simulink model "tqdtqr_rebuild_V3"  (R2021b)
settings: Solver=VariableStepAuto  StartTime=0.0  StopTime=10.0  RelTol=1e-3
undefined symbols (not defined in the file): ATQD_AfterTqMinGain_X_Deg, ATQD_APSCreepBaseTqD_X_kph, ATQD_APSCreepBaseTqD_Y_Deg, ATQD_APSCreepBaseTqR_X_kph, ATQD_APSCreepBaseTqR_Y_Deg, ATQD_APSCreepIterm_X_kph, ATQD_APSCreepIterm_Y_kph, ATQD_APSCreepPterm_X_kph, ATQD_APSCreepPterm_Y_kph, ATQD_APSDecReq_X_kph, ATQD_APSDecReq_Y_mps2, ATQD_APSDecReqCMD_X_kph, ATQD_APSDecReqTs_X_pct, ATQD_APSDecTimeGain_X_Deg, ATQD_APSDecTimeGain_Y_s, ATQD_APSReqLowSpd_X_Deg, ATQD_AutoHoldReleaseBPS_X_Deg, ATQD_AWDLoadTrqnsGain_X_kg, ATQD_AWDLoadTrqnsGain_Y_pct, ATQD_BOSEnBPSPosn_X_kph, ATQD_BOSMap_X_rpm, ATQD_BOSMap_Y_pct, ATQD_CreepBaseTqD_X_kph, ATQD_CreepBaseTqD_Y_Deg, ATQD_CreepBaseTqR_X_kph, ATQD_CreepBaseTqR_Y_Deg, ATQD_CreepBPSDisPosn_X_Deg, ATQD_CreepBPSDisPosnR_X_Deg, ATQD_CreepBPSEnPosn_X_Deg, ATQD_CreepBPSEnPosnR_X_Deg, ATQD_CreepDeltaTq_X_kph, ATQD_CreepIterm_X_kph, ATQD_CreepIterm_Y_kph, ATQD_CreepItermMaxLimit_X_pct, ATQD_CreepPreloadTime_X_kph, ATQD_CreepPreloadTq_X_kph, ATQD_CreepPreloadTq_Y_s, ATQD_CreepProtTq_X_Deg, ATQD_CreepPterm_X_kph, ATQD_CreepPterm_Y_kph, ATQD_CreepRrTqSpRat_X_rpm, ATQD_CreepRrTqSpRat_Y_Nm, ATQD_CreepTargetSpdD_X_pct, ATQD_CreepTargetSpdR_X_pct, ATQD_CreepUpLimitTq_X_rpm, ATQD_DecIneOPDHoldEnDelay_X_Deg, ATQD_DecIneOPDHoldEnDelay_Y_bar, ATQD_ECOTqMapD_X_rpm, ATQD_ECOTqMapD_Y_pct, ATQD_EMTqMapD_X_rpm, ATQD_EMTqMapD_Y_pct, ATQD_EOPDTqMapDCon_X_rpm, ATQD_EOPDTqMapDCon_Y_Deg, ATQD_EstInitVehWeight_X_c, ATQD_FAfterTqCMDGain_X_rpm, ATQD_FAfterTqCMDGain_Y_pct, ATQD_ForceLowSpd_X_Deg, ATQD_ForcePLimitSpd_X_Deg, ATQD_FrLossMAPLowV_X_rpm, ATQD_FrLossMAPLowV_Y_Nm ... (+949)
libraries: simulink x235, hcu_lib x208, tqr x63, tqd x6
(part 9 of 37)

== system tqdtqr_rebuild_V3/Input_Convert/Main function/Add B regen to ramp enable judge ==
  note: Rear B regen
  note: Front B regen
  BSCPIn_outputs : Inport
  BSignalConvert_outputs : Inport  Port=2
  BFunction_outputs : Inport  Port=3
  AND{6..7,10,12} (4 alike) : Logic  AllPortsSameDT=off  OutDataTypeStr=boolean
  AND{8..9,11,13} (4 alike) : Logic  Operator=OR  AllPortsSameDT=off  OutDataTypeStr=boolean
  AND{3,5,14,16} (4 alike) : Logic  Inputs=3  AllPortsSameDT=off  OutDataTypeStr=boolean
  AND15 : Logic  Operator=OR  Inputs=3  AllPortsSameDT=off  OutDataTypeStr=boolean
  AND17 : Logic  Operator=OR  Inputs=3  AllPortsSameDT=off  OutDataTypeStr=boolean
  Add2 : Sum
  Add3 : Sum
  Bus Selector : BusSelector  OutputSignals=task_time_s,VVMC_ADASActive_flg,VINP_FrntAxlTrqReqBrk_Nm,VINP_FrRBCActive_flg,VINP_RearAxlTrqReqBrk_Nm,VINP_RrRBCActive_flg
  Bus Selector1 : BusSelector  OutputSignals=VTQD_BrkSwSta_flg,VTQR_RampTqCMDGain_c
  Bus Selector2 : BusSelector  OutputSignals=VTQD_GearActualPosn_enum
  Constant14 : Constant  Value=ONE_INT
  Constant15 : Constant  Value=KTQR_NewRampArchSW_flg
  Constant22 : Constant  Value=ONE_INT
  Constant23 : Constant  Value=ENUM_GEARACTUALPOSN_R
  Constant30 : Constant  Value=KTQR_NewRampArchSW_flg
  Constant31 : Constant  Value=ENUM_GEARACTUALPOSN_R
  Constant32 : Constant  Value=KTQR_ACCCancelNoRBC_flg
  Constant33 : Constant  Value=KTQR_ACCCancelNoRBC_flg
  Constant{4..5,34,39} (4 alike) : Constant  Value=ZERO_FLOAT
  Constant35 : Constant  Value=KTQR_ADASCancelBRgnSlopeF_Nmps
  Constant{36..38,41} (4 alike) : Constant  Value=KTQR_ADASCancelBRgnSlopeSW_flg
  Constant40 : Constant  Value=KTQR_ADASCancelBRgnSlopeR_Nmps
  Detect Decrease{,1..3} (4 alike) : simulink/Logic and Bit Operations/Detect Decrease  vinit=0.0  OutDataTypeStr=boolean
  Divide : Product  Inputs=**
  Divide1 : Product  Inputs=**
  Equal8 : RelationalOperator  Operator===  OutDataTypeStr=boolean  RndMeth=Simplest
  Equal9 : RelationalOperator  Operator===  OutDataTypeStr=boolean  RndMeth=Simplest
  NOT{,1..11} (12 alike) : Logic  Operator=NOT  AllPortsSameDT=off  OutDataTypeStr=boolean
  Product2 : Product
  Product5 : Product
  Relational Operator : RelationalOperator  Operator=<=  OutDataTypeStr=boolean  RndMeth=Simplest
  Relational Operator1 : RelationalOperator  Operator=<=  OutDataTypeStr=boolean  RndMeth=Simplest
  SR_Latch{1..4} (4 alike) : hcu_lib/Basic_Blocks/SR_Latch
  Switch{4..5,12,17,22..27} (10 alike) : Switch  Criteria=u2 ~= 0
      settings: AttributesFormatString=%<Criteria>
  Unit Delay{,1..3} (4 alike) : UnitDelay  InitialCondition=single(0)  SampleTime=-1  HasFrameUpgradeWarning=on
      settings: AttributesFormatString=%<InitialCondition>
  VTQD_FEDUWhlTqBRegen_Nm : Outport
  VTQD_REDUWhlTqBRegen_Nm : Outport  Port=2
  wires:
  [VTQD_BrkSwSta_flg] -> AND14/2
  [task_time_s] -> Divide/2
  [VVMC_ADASActive_flg] -> Detect Decrease2/1
  Constant36/1 -> AND14/3
  Divide/1 -> Add2/2
  [VINP_FrRBCActive_flg] -> NOT9/1
  SR_Latch3/1 -> [VTQR_ADASCancelBRgnRampF_flg]  "VTQR_ADASCancelBRgnRampF_flg"
  [VTQD_BrkSwSta_flg] -> NOT8/1
  [VTQR_FrntAxlTrqReqBrkRamp_Nm] -> Unit Delay2/1
  [VINP_FrntAxlTrqReqBrk_Nm] -> Relational Operator/2
  Unit Delay2/1 -> Relational Operator/1
  NOT8/1 -> AND15/2
  [VTQR_ADASCancelBRgnRampF_flg] -> Switch22/2
  Detect Decrease2/1 -> AND14/1
  Unit Delay/1 -> Add2/1
  AND14/1 -> SR_Latch3/1
  AND15/1 -> SR_Latch3/2
  Relational Operator/1 -> AND15/1
  Switch22/1 -> Unit Delay/1, [VTQR_FrntAxlTrqReqBrkRamp_Nm]  "VTQR_FrntAxlTrqReqBrkRamp_Nm"
  Constant35/1 -> Divide/1
  Constant34/1 -> Switch22/3
  Add2/1 -> Switch22/1
  NOT9/1 -> AND15/3
  [VINP_FrRBCActive_flg] -> AND3/3
  [VVMC_ADASActive_flg] -> NOT1/1
  [VINP_FrntAxlTrqReqBrk_Nm] -> Switch26/3
  [VTQR_RampTqCMDGain_c] -> Switch12/1
  NOT1/1 -> AND3/1
  Switch26/1 -> Switch23/1
  AND13/1 -> SR_Latch2/2
  NOT3/1 -> AND8/2
  Constant30/1 -> AND7/2
  AND12/1 -> SR_Latch2/1
  [VVMC_ADASActive_flg] -> Detect Decrease1/1
  [VTQD_BrkSwSta_flg] -> NOT5/1
  AND3/1 -> Switch4/2
  AND7/1 -> Switch12/2
  AND8/1 -> AND3/2
  Equal9/1 -> AND7/1
  Constant31/1 -> Equal9/2
  Constant4/1 -> Switch4/3
  Constant32/1 -> NOT3/1
  [VTQD_GearActualPosn_enum] -> Equal9/1
  [VTQR_FrntAxlTrqReqBrkRamp_Nm] -> Switch26/1
  SR_Latch2/1 -> NOT7/1
  [VTQR_ADASCancelBRgnRampF_flg] -> Switch26/2
  [VINP_FrntAxlTrqReqBrk_Nm] -> Switch23/3
  Switch23/1 -> Switch4/1
  [VVMC_ADASActive_flg] -> AND13/1
  [VTQD_BrkSwSta_flg] -> AND13/2
  Detect Decrease1/1 -> AND12/1
  Switch12/1 -> Product2/2
  NOT5/1 -> AND12/2
  Switch4/1 -> Product2/1
  Constant37/1 -> Switch23/2
  NOT7/1 -> AND8/1
  Constant14/1 -> Switch12/3
  BSCPIn_outputs/1 -> Bus Selector/1
  Bus Selector/2 -> [VVMC_ADASActive_flg]  "<VVMC_ADASActive_flg>"
  Bus Selector/3 -> [VINP_FrntAxlTrqReqBrk_Nm]  "<VINP_FrntAxlTrqReqBrk_Nm>"
  Bus Selector/4 -> [VINP_FrRBCActive_flg]  "<VINP_FrRBCActive_flg>"
  Bus Selector/1 -> [task_time_s]  "<task_time_s>"
  BSignalConvert_outputs/1 -> Bus Selector1/1
  BFunction_outputs/1 -> Bus Selector2/1
  Bus Selector1/1 -> [VTQD_BrkSwSta_flg]  "<VTQD_BrkSwSta_flg>"
  Bus Selector2/1 -> [VTQD_GearActualPosn_enum]  "<VTQD_GearActualPosn_enum>"
  Bus Selector1/2 -> [VTQR_RampTqCMDGain_c]  "<VTQR_RampTqCMDGain_c>"
  Product2/1 -> [VTQD_FEDUWhlTqBRegen_Nm]  "VTQD_FEDUWhlTqBRegen_Nm"
  [VTQD_FEDUWhlTqBRegen_Nm] -> VTQD_FEDUWhlTqBRegen_Nm/1
  Relational Operator1/1 -> AND17/1
  [VINP_RrRBCActive_flg] -> NOT11/1
  [VINP_RearAxlTrqReqBrk_Nm] -> Relational Operator1/2
  Detect Decrease3/1 -> AND16/1
  [VTQD_BrkSwSta_flg] -> NOT10/1
  Divide1/1 -> Add3/2
  [VVMC_ADASActive_flg] -> Detect Decrease3/1
  [VTQR_ADASCancelBRgnRampR_flg] -> Switch25/2
  Switch25/1 -> Unit Delay1/1, [VTQR_RearAxlTrqReqBrkRamp_Nm]  "VTQR_RearAxlTrqReqBrkRamp_Nm"
  Unit Delay3/1 -> Relational Operator1/1
  AND17/1 -> SR_Latch4/2
  [VTQR_RearAxlTrqReqBrkRamp_Nm] -> Unit Delay3/1
  NOT11/1 -> AND17/3
  NOT10/1 -> AND17/2
  Add3/1 -> Switch25/1
  SR_Latch4/1 -> [VTQR_ADASCancelBRgnRampR_flg]  "VTQR_ADASCancelBRgnRampR_flg"
  Unit Delay1/1 -> Add3/1
  Constant39/1 -> Switch25/3
  Constant41/1 -> AND16/3
  Constant40/1 -> Divide1/1
  [VTQD_BrkSwSta_flg] -> AND16/2
  AND16/1 -> SR_Latch4/1
  [task_time_s] -> Divide1/2
  Constant22/1 -> Switch17/3
  [VTQR_RampTqCMDGain_c] -> Switch17/1
  [VVMC_ADASActive_flg] -> NOT2/1
  AND5/1 -> Switch5/2
  NOT2/1 -> AND5/1
  Constant5/1 -> Switch5/3
  [VVMC_ADASActive_flg] -> Detect Decrease/1
  Switch5/1 -> Product5/1
  [VINP_RearAxlTrqReqBrk_Nm] -> Switch24/3
  [VINP_RrRBCActive_flg] -> AND5/3
  [VTQR_RearAxlTrqReqBrkRamp_Nm] -> Switch27/1
  [VTQD_BrkSwSta_flg] -> NOT/1
  [VTQD_BrkSwSta_flg] -> AND11/2
  Detect Decrease/1 -> AND10/1
  [VTQD_GearActualPosn_enum] -> Equal8/1
  AND10/1 -> SR_Latch1/1
  Constant15/1 -> AND6/2
  Equal8/1 -> AND6/1
  Switch17/1 -> Product5/2
  AND11/1 -> SR_Latch1/2
  [VTQR_ADASCancelBRgnRampR_flg] -> Switch27/2
  Switch27/1 -> Switch24/1
  Constant23/1 -> Equal8/2
  [VINP_RearAxlTrqReqBrk_Nm] -> Switch27/3
  Constant38/1 -> Switch24/2
  NOT4/1 -> AND9/2
  AND6/1 -> Switch17/2
  NOT6/1 -> AND9/1
  Constant33/1 -> NOT4/1
  [VVMC_ADASActive_flg] -> AND11/1
  NOT/1 -> AND10/2
  SR_Latch1/1 -> NOT6/1
  AND9/1 -> AND5/2
  Switch24/1 -> Switch5/1
  Product5/1 -> [VTQD_REDUWhlTqBRegen_Nm]  "VTQD_REDUWhlTqBRegen_Nm"
  [VTQD_REDUWhlTqBRegen_Nm] -> VTQD_REDUWhlTqBRegen_Nm/1
  Bus Selector/5 -> [VINP_RearAxlTrqReqBrk_Nm]  "<VINP_RearAxlTrqReqBrk_Nm>"
  Bus Selector/6 -> [VINP_RrRBCActive_flg]  "<VINP_RrRBCActive_flg>"

== system tqdtqr_rebuild_V3/Input_Convert/Main function/AvaliableTqLimit function ==
  BSCPIn_outputs : Inport
  BSignalConvert_outputs : Inport  Port=2
  BFunction_outputs : Inport  Port=3
  BMain_outputs : Inport  Port=4
  VTQD_IVIRockModeEn_flg : Inport  Port=5
  VTQD_FrEDUSpRat_rat : Inport  Port=6
  VTQD_RrEDUSpRat_rat : Inport  Port=7
  Bus Selector : BusSelector  OutputSignals=task_time_s,VINP_HVBPwrAvailDchrg_kW,VINP_HVBPwrAvailChrg_kW,VINP_FrMotorAvailTq_Nm,VINP_RrMotorAvailTq_Nm,VINP_FrRegenAvailTq_Nm,VINP_RrRegenAvailTq_Nm,VINP_VehicleType_enum,VINP_FrMCUDCBusVolt_V,VINP_RrMCUDCBusVolt_V,VPMM_DrivetrainSelect_enum,VINP_FrMCUTemp_C,VINP_FrTMTemp_C,VINP_RrMCUTemp_C,VINP_RrTMTemp_C,VVMC_EstSlope_Deg,VINP_FrPTCSActive_flg,VINP_RrPTCSActive_flg,VTQD_ActAPSPosn_pct
  Bus Selector1 : BusSelector  OutputSignals=VTQD_FrShaftSpd_rpm,VTQD_RrShaftSpd_rpm
  Bus Selector2 : BusSelector  OutputSignals=VTQD_GearActualPosn_enum,VTQD_FrontSlideRate_pct,VTQD_RearSlideRate_pct
  Bus Selector4 : BusSelector  OutputSignals=VTQD_CoordWhlTqDemFr_Nm,VTQD_CoordWhlTqDemRr_Nm
  Constant2 : Constant  Value=KTQD_FrBatapCont_factor
  Constant{27,30,51..52} (4 alike) : Constant  Value=ONE_FLOAT
  Constant28 : Constant  Value=KTQD_FAfterTqCMDGainInc_c
  Constant29 : Constant  Value=KTQD_FAfterTqCMDGainDec_c
  Constant31 : Constant  Value=KTQD_RAfterTqCMDGainInc_c
  Constant32 : Constant  Value=KTQD_RAfterTqCMDGainDec_c
  Constant5 : Constant  Value=KTQD_RrBatapCont_factor
  MTQD_AfterTqMinGain_Y_c : Lookup_n-D  NumberOfTableDimensions=1  BreakpointsForDimension1=ATQD_AfterTqMinGain_X_Deg  Table=MTQD_AfterTqMinGain_Y_c  InternalRulePriority=Speed  RndMeth=Simplest  InputSameDT=on
  MTQD_FAfterTqCMDGain_Z_c : Lookup_n-D  BreakpointsForDimension1=ATQD_FAfterTqCMDGain_Y_pct  BreakpointsForDimension2=ATQD_FAfterTqCMDGain_X_rpm  Table=MTQD_FAfterTqCMDGain_Z_c  InternalRulePriority=Speed  RndMeth=Simplest  InputSameDT=on
      settings: InputPortMap=u0,u1
  MTQD_RAfterTqCMDGain_Z_c : Lookup_n-D  BreakpointsForDimension1=ATQD_FAfterTqCMDGain_Y_pct  BreakpointsForDimension2=ATQD_FAfterTqCMDGain_X_rpm  Table=MTQD_RAfterTqCMDGain_Z_c  InternalRulePriority=Speed  RndMeth=Simplest  InputSameDT=on
      settings: InputPortMap=u0,u1
  Max2 : MinMax  Function=max  Inputs=2
  Max3 : MinMax  Function=max  Inputs=2
  RateLimit : hcu_lib/Basic_Blocks/RateLimit
  RateLimit1 : hcu_lib/Basic_Blocks/RateLimit
  Switch13 : Switch  Criteria=u2 > Threshold
  Switch14 : Switch  Criteria=u2 > Threshold
  TorqueCapacityCalcalation : Subsystem
  VTQD_WhlTqCapMotFr_Nm : Outport
  VTQD_WhlTqCapMotRr_Nm : Outport  Port=2
  VTQD_WhlTqCapGenFr_Nm : Outport  Port=3
  VTQD_WhlTqCapGenRr_Nm : Outport  Port=4
  VTQD_MotorLossTotal_kw : Outport  Port=5
  VTQD_FAfterTqCMDGain_c : Outport  Port=6
  VTQD_RAfterTqCMDGain_c : Outport  Port=7
  wires:
  TorqueCapacityCalcalation/5(VTQD_MotorLossTotal_kw) -> [VTQD_MotorLossTotal_kw]
  [VINP_RrMCUTemp_C] -> TorqueCapacityCalcalation/22(VINP_RrMCUTemp_C)
  TorqueCapacityCalcalation/3(VTQD_WhlTqCapGenFr_Nm) -> [VTQD_WhlTqCapGenFr_Nm]
  [VINP_FrTMTemp_C] -> TorqueCapacityCalcalation/21(VINP_FrTMTemp_C)
  [VINP_FrMCUTemp_C] -> TorqueCapacityCalcalation/20(VINP_FrMCUTemp_C)
  [VPMM_DrivetrainSelect_enum] -> TorqueCapacityCalcalation/19(VPMM_DrivetrainSelect_enum)
  [VTQD_CoordWhlTqDemFr_Nm] -> TorqueCapacityCalcalation/15(VTQD_CoordWhlTqDemFr_Nm)
  [VTQD_RrEDUSpRat_rat] -> TorqueCapacityCalcalation/8(VTQD_RrEDUSpRat_rat)
  [VINP_FrRegenAvailTq_Nm] -> TorqueCapacityCalcalation/11(VINP_FrRegenAvailTq_Nm)
  Constant5/1 -> TorqueCapacityCalcalation/6(KTQD_RrBatapCont_factor)
  Constant2/1 -> TorqueCapacityCalcalation/5(KTQD_FrBatapCont_factor)
  [VINP_RrTMTemp_C] -> TorqueCapacityCalcalation/23(VINP_RrTMTemp_C)
  TorqueCapacityCalcalation/1(VTQD_WhlTqCapMotFr_Nm) -> [VTQD_WhlTqCapMotFr_Nm]
  [VTQD_CoordWhlTqDemRr_Nm] -> TorqueCapacityCalcalation/16(VTQD_CoordWhlTqDemRr_Nm)
  [VINP_FrMCUDCBusVolt_V] -> TorqueCapacityCalcalation/17(VINP_FrMCUDCBusVolt_V)
  [VINP_RrMotorAvailTq_Nm] -> TorqueCapacityCalcalation/10(VINP_RrMotorAvailTq_Nm)
  [VTQD_GearActualPosn_enum] -> TorqueCapacityCalcalation/13(VTQD_GearActualPosn_enum)
  [VINP_FrMotorAvailTq_Nm] -> TorqueCapacityCalcalation/9(VINP_FrMotorAvailTq_Nm)
  [VTQD_RrShaftSpd_rpm] -> TorqueCapacityCalcalation/2(VTQD_RrShaftSpd_rpm)
  [VINP_VehicleType_enum] -> TorqueCapacityCalcalation/14(VINP_VehicleType_enum)
  TorqueCapacityCalcalation/4(VTQD_WhlTqCapGenRr_Nm) -> [VTQD_WhlTqCapGenRr_Nm]
  [VINP_RrRegenAvailTq_Nm] -> TorqueCapacityCalcalation/12(VINP_RrRegenAvailTq_Nm)
  [VTQD_FrShaftSpd_rpm] -> TorqueCapacityCalcalation/1(VTQD_FrShaftSpd_rpm)
  TorqueCapacityCalcalation/2(VTQD_WhlTqCapMotRr_Nm) -> [VTQD_WhlTqCapMotRr_Nm]
  [VINP_HVBPwrAvailDchrg_kw] -> TorqueCapacityCalcalation/3(VINP_HVBPwrAvailDchrg_kw)
  [VINP_RrMCUDCBusVolt_V] -> TorqueCapacityCalcalation/18(VINP_RrMCUDCBusVolt_V)
  [VTQD_FrEDUSpRat_rat] -> TorqueCapacityCalcalation/7(VTQD_FrEDUSpRat_cmd)
  [VINP_HVBPwrAvailChrg_kw] -> TorqueCapacityCalcalation/4(VINP_HVBPwrAvailChrg_kw)
  BSCPIn_outputs/1 -> Bus Selector/1
  BSignalConvert_outputs/1 -> Bus Selector1/1
  BFunction_outputs/1 -> Bus Selector2/1
  Bus Selector1/1 -> [VTQD_FrShaftSpd_rpm]  "<VTQD_FrShaftSpd_rpm>"
  Bus Selector1/2 -> [VTQD_RrShaftSpd_rpm]  "<VTQD_RrShaftSpd_rpm>"
  Bus Selector/2 -> [VINP_HVBPwrAvailDchrg_kw]  "<VINP_HVBPwrAvailDchrg_kW>"
  Bus Selector/3 -> [VINP_HVBPwrAvailChrg_kw]  "<VINP_HVBPwrAvailChrg_kW>"
  Bus Selector/4 -> [VINP_FrMotorAvailTq_Nm]  "<VINP_FrMotorAvailTq_Nm>"
  Bus Selector/5 -> [VINP_RrMotorAvailTq_Nm]  "<VINP_RrMotorAvailTq_Nm>"
  Bus Selector/6 -> [VINP_FrRegenAvailTq_Nm]  "<VINP_FrRegenAvailTq_Nm>"
  Bus Selector/7 -> [VINP_RrRegenAvailTq_Nm]  "<VINP_RrRegenAvailTq_Nm>"
  Bus Selector2/1 -> [VTQD_GearActualPosn_enum]  "<VTQD_GearActualPosn_enum>"
  Bus Selector/8 -> [VINP_VehicleType_enum]  "<VINP_VehicleType_enum>"
  BMain_outputs/1 -> Bus Selector4/1
  Bus Selector4/1 -> [VTQD_CoordWhlTqDemFr_Nm]  "<VTQD_CoordWhlTqDemFr_Nm>"
  Bus Selector4/2 -> [VTQD_CoordWhlTqDemRr_Nm]  "<VTQD_CoordWhlTqDemRr_Nm>"
  Bus Selector/1 -> [task_time_s]  "<task_time_s>"
  Bus Selector/9 -> [VINP_FrMCUDCBusVolt_V]  "<VINP_FrMCUDCBusVolt_V>"
  Bus Selector/10 -> [VINP_RrMCUDCBusVolt_V]  "<VINP_RrMCUDCBusVolt_V>"
  Bus Selector/11 -> [VPMM_DrivetrainSelect_enum]  "<VPMM_DrivetrainSelect_enum>"
  Bus Selector/12 -> [VINP_FrMCUTemp_C]  "<VINP_FrMCUTemp_C>"
  Bus Selector/13 -> [VINP_FrTMTemp_C]  "<VINP_FrTMTemp_C>"
  Bus Selector/14 -> [VINP_RrMCUTemp_C]  "<VINP_RrMCUTemp_C>"
  Bus Selector/15 -> [VINP_RrTMTemp_C]  "<VINP_RrTMTemp_C>"
  Switch13/1 -> Max2/1
  [VTQD_FrShaftSpd_rpm] -> MTQD_FAfterTqCMDGain_Z_c/2
  Constant51/1 -> Switch13/1
  [task_time_s] -> RateLimit/3
  [VINP_FrPTCSActive_flg] -> Switch13/2
  [VTQD_AfterTqMinGain_c] -> Switch13/3
  MTQD_FAfterTqCMDGain_Z_c/1 -> Max2/2
  Constant29/1 -> RateLimit/5
  Max2/1 -> RateLimit/1
  Constant27/1 -> RateLimit/2
  RateLimit/1 -> [VTQD_FAfterTqCMDGain_c]  "VTQD_FAfterTqCMDGain_c"
  Constant28/1 -> RateLimit/4
  [VTQD_FrontSlideRate_pct] -> MTQD_FAfterTqCMDGain_Z_c/1
  [VTQD_RearSlideRate_pct] -> MTQD_RAfterTqCMDGain_Z_c/1
  Constant30/1 -> RateLimit1/2
  [VINP_RrPTCSActive_flg] -> Switch14/2
  MTQD_RAfterTqCMDGain_Z_c/1 -> Max3/2
  Constant32/1 -> RateLimit1/5
  Constant31/1 -> RateLimit1/4
  Switch14/1 -> Max3/1
  [VTQD_RrShaftSpd_rpm] -> MTQD_RAfterTqCMDGain_Z_c/2
  [VTQD_AfterTqMinGain_c] -> Switch14/3
  Constant52/1 -> Switch14/1
  RateLimit1/1 -> [VTQD_RAfterTqCMDGain_c]  "VTQD_RAfterTqCMDGain_c"
  Max3/1 -> RateLimit1/1
  [task_time_s] -> RateLimit1/3
  [VVMC_EstSlope_Deg] -> MTQD_AfterTqMinGain_Y_c/1
  MTQD_AfterTqMinGain_Y_c/1 -> [VTQD_AfterTqMinGain_c]  "VTQD_AfterTqMinGain_c"
  Bus Selector/16 -> [VVMC_EstSlope_Deg]  "<VVMC_EstSlope_Deg>"
  Bus Selector/17 -> [VINP_FrPTCSActive_flg]  "<VINP_FrPTCSActive_flg>"
  Bus Selector2/2 -> [VTQD_FrontSlideRate_pct]  "<VTQD_FrontSlideRate_pct>"
  Bus Selector/18 -> [VINP_RrPTCSActive_flg]  "<VINP_RrPTCSActive_flg>"
  Bus Selector2/3 -> [VTQD_RearSlideRate_pct]  "<VTQD_RearSlideRate_pct>"
  [VTQD_WhlTqCapMotFr_Nm] -> VTQD_WhlTqCapMotFr_Nm/1
  [VTQD_WhlTqCapMotRr_Nm] -> VTQD_WhlTqCapMotRr_Nm/1
  [VTQD_WhlTqCapGenFr_Nm] -> VTQD_WhlTqCapGenFr_Nm/1
  [VTQD_RAfterTqCMDGain_c] -> VTQD_RAfterTqCMDGain_c/1
  VTQD_FrEDUSpRat_rat/1 -> [VTQD_FrEDUSpRat_rat]
  VTQD_RrEDUSpRat_rat/1 -> [VTQD_RrEDUSpRat_rat]
  [VTQD_WhlTqCapGenRr_Nm] -> VTQD_WhlTqCapGenRr_Nm/1
  [VTQD_MotorLossTotal_kw] -> VTQD_MotorLossTotal_kw/1
  [VTQD_FAfterTqCMDGain_c] -> VTQD_FAfterTqCMDGain_c/1
  [VTQD_IVIRockModeEn_flg] -> TorqueCapacityCalcalation/24(VTQD_IVIRockModeEn_flg)
  [VTQD_ActAPSPosn_pct] -> TorqueCapacityCalcalation/25(VTQD_ActAPSPosn_pct)
  [task_time_s] -> TorqueCapacityCalcalation/26(task_time_s)
  Bus Selector/19 -> [VTQD_ActAPSPosn_pct]  "<VTQD_ActAPSPosn_pct>"
  VTQD_IVIRockModeEn_flg/1 -> [VTQD_IVIRockModeEn_flg]

== system tqdtqr_rebuild_V3/Input_Convert/Main function/DriverWhlTqDem function ==
  BSCPIn_outputs : Inport
  BSignalConvert_outputs : Inport  Port=2
  BFunction_outputs : Inport  Port=3
  BMain_outputs : Inport  Port=4
  VTQD_TqSourceFr_enum : Inport  Port=5
  VTQD_TqSourceRr_enum : Inport  Port=6
  VTQR_FShaftSpdTqLimLow_flg : Inport  Port=7
  VTQR_FTimerTqLimLow_flg : Inport  Port=8
  VTQR_RShaftSpdTqLimLow_flg : Inport  Port=9
  VTQR_RTimerTqLimLow_flg : Inport  Port=10
  BOS : Subsystem
  Creep : Subsystem
  Driver mode determination : Subsystem
  Low speed control : Subsystem
  Pedal G-Control Mode : Subsystem
  PedalMapWhlTq : Subsystem
  Preload system : Subsystem
  "Rock Mode torque " : Subsystem
  RollingRegenJudge : Subsystem
  VTQD_RollRegenEnable_flg : Outport
  VTQD_BOSEnable_flg : Outport  Port=2
  VTQD_BOSTq_Nm : Outport  Port=3
  VTQD_IVIRockModeEn_flg : Outport  Port=4
  VTQD_LoSpdBrkCtrl_flg : Outport  Port=5
  VTQD_RockModeTCSReq_flg : Outport  Port=6
  VTQD_RockModePedTq_Nm : Outport  Port=7
  VTQD_RockModeTqLim_flg : Outport  Port=8
  VTQD_PreLoadPreEn_flg : Outport  Port=9
  VTQD_PreloadTq_Nm : Outport  Port=10
  VTQD_PreLoadHold_flg : Outport  Port=11
  VTQD_CreepWhlTqDem_Nm : Outport  Port=12
  VTQD_CreepPrLoadEnable_flg : Outport  Port=13
  VTQD_CreepProtTqEn_flg : Outport  Port=14
  VTQD_PedalMapWhlTq_Nm : Outport  Port=15
  VTQD_EVDriveModeValid_flg : Outport  Port=16
  VTQD_RegenTqLimitEn_flg : Outport  Port=17
  VTQD_PedAccTqEn_flg : Outport  Port=18
  VTQD_SlideRegenLimTq_Nm : Outport  Port=19
  VTQD_OPDOn2Off_flg : Outport  Port=20
  VTQD_CreepTCSActive_flg : Outport  Port=21
  VTQD_FrPreloadTq_Nm : Outport  Port=22
  VTQD_RrPreloadTq_Nm : Outport  Port=23
  VTQD_CreepEnable_flg : Outport  Port=24
  VTQD_CreepBaseTqD_Nm : Outport  Port=25
  wires:
  BFunction_outputs/1 -> [BFunction_outputs]
  BSignalConvert_outputs/1 -> [BSignalConvert_outputs]
  [VTQD_CreepEnable_flg] -> Driver mode determination/7(VTQD_CreepEnable_flg)
  [VTQD_RollRegenEnable_flg] -> Driver mode determination/4(VTQD_RollRegenEnable_flg)
  [VTQD_RollingShaftSpd_rpm] -> Driver mode determination/5(VTQD_RollingShaftSpd_rpm)
  [VTQD_CreepEnable_flg] -> RollingRegenJudge/5(VTQD_CreepEnable_flg)
  RollingRegenJudge/1(VTQD_RollRegenEnable_flg) -> [VTQD_RollRegenEnable_flg]
  RollingRegenJudge/2(VTQD_RollingShaftSpd_rpm) -> [VTQD_RollingShaftSpd_rpm]
  [VTQD_PedalMapWhlTq_Nm] -> Creep/4(VTQD_PedalMapWhlTq_Nm)
  [VTQD_PedAccTqEn_flg] -> Creep/7(VTQD_PedAccTqEn_flg)
  [VTQD_PreLoadPreEn_flg] -> Creep/6(VTQD_PreLoadPreEn_flg)
  [VTQD_LoSpdBrkCtrl_flg] -> Creep/5(VTQD_LoSpdBrkCtrl_flg)
  Driver mode determination/1(VTQD_PedalMapWhlTqMerge_Nm) -> [VTQD_PedalMapWhlTqMerge_Nm]
  BSCPIn_outputs/1 -> [BSCPIn_outputs]
  [BSCPIn_outputs] -> RollingRegenJudge/1(BSCPIn_outputs)
  [BSignalConvert_outputs] -> RollingRegenJudge/2(BSignalConvert_outputs)
  [BSCPIn_outputs] -> Driver mode determination/1(BSCPIn_outputs)
  [BSignalConvert_outputs] -> Driver mode determination/2(BSignalConvert_outputs)
  [BFunction_outputs] -> Driver mode determination/3(BFunction_outputs)
  [BSCPIn_outputs] -> Creep/1(BSCPIn_outputs)
  [BSignalConvert_outputs] -> Creep/2(BSignalConvert_outputs)
  [BFunction_outputs] -> Creep/3(BFunction_outputs)
  [BSCPIn_outputs] -> Pedal G-Control Mode/1(BSCPIn_outputs)
  [BSignalConvert_outputs] -> Pedal G-Control Mode/2(BSignalConvert_outputs)
  [BFunction_outputs] -> Pedal G-Control Mode/3(BFunction_outputs)
  Pedal G-Control Mode/1(VTQD_PedAccTqEn_flg) -> [VTQD_PedAccTqEn_flg]
  Pedal G-Control Mode/2(VTQD_PedalTqCal_Nm) -> [VTQD_PedalTqCal_Nm]
  [BSCPIn_outputs] -> PedalMapWhlTq/1(BSCPIn_outputs)
  [BSignalConvert_outputs] -> PedalMapWhlTq/2(BSignalConvert_outputs)
  [VTQD_PedAccTqEn_flg] -> PedalMapWhlTq/3(VTQD_PedAccTqEn_flg)
  [VTQD_PedalTqCal_Nm] -> PedalMapWhlTq/4(VTQD_PedalTqCal_Nm)
  [VTQD_PedalMapWhlTqMerge_Nm] -> PedalMapWhlTq/5(VTQD_PedalMapWhlTqMerge_Nm)
  [VTQD_CreepPrLoadEnable_flg] -> Pedal G-Control Mode/4(VTQD_CreepPrLoadEnable_flg)
  PedalMapWhlTq/1(VTQD_PedalMapWhlTq_Nm) -> [VTQD_PedalMapWhlTq_Nm]
  PedalMapWhlTq/2(VTQD_PreDecTqLowLim_Nm) -> [VTQD_PreDecTqLowLim_Nm]
  [VTQD_PreDecTqLowLim_Nm] -> Driver mode determination/8(VTQD_PreDecTqLowLim_Nm)
  Creep/1(VTQD_CreepEnable_flg) -> [VTQD_CreepEnable_flg]
  Creep/2(VTQD_CreepWhlTqDem_Nm) -> [VTQD_CreepWhlTqDem_Nm]  "VTQD_CreepWhlTqDem_Nm"
  Creep/3(VTQD_CreepPrLoadEnable_flg) -> [VTQD_CreepPrLoadEnable_flg]
  Creep/4(VTQD_OPDOn2Off_flg) -> [VTQD_OPDOn2Off_flg]
  Creep/5(VTQD_CreepProtTqEn_flg) -> [VTQD_CreepProtTqEn_flg]
  Creep/6(VTQD_CreepBaseTqD_Nm) -> [VTQD_CreepBaseTqD_Nm]
  Creep/7(VTQD_CreepBaseTqR_Nm) -> [VTQD_CreepBaseTqR_Nm]
  Creep/8(VTQD_HighBPSPosn_flg) -> [VTQD_HighBPSPosn_flg]
  Creep/9(VTQD_CreepTCSActive_flg) -> [VTQD_CreepTCSActive_flg]
  [BSCPIn_outputs] -> BOS/1(BSCPIn_outputs)
  [BSignalConvert_outputs] -> BOS/2(BSignalConvert_outputs)
  [BFunction_outputs] -> BOS/3(BFunction_outputs)
  [VTQD_PedalMapWhlTq_Nm] -> BOS/4(VTQD_PedalMapWhlTq_Nm)
  [VTQD_CreepBaseTqR_Nm] -> BOS/5(VTQD_CreepBaseTqR_Nm)
  [VTQD_CreepBaseTqD_Nm] -> BOS/6(VTQD_CreepBaseTqD_Nm)
  [VTQD_HighBPSPosn_flg] -> BOS/7(VTQD_HighBPSPosn_flg)
  BOS/1(VTQD_BOSEnable_flg) -> [VTQD_BOSEnable_flg]
  BOS/2(VTQD_BOSTq_Nm) -> [VTQD_BOSTq_Nm]
  Driver mode determination/2(VTQD_EVDriveModeValid_flg) -> [VTQD_EVDriveModeValid_flg]
  PedalMapWhlTq/3(VTQD_RegenTqLimitEn_flg) -> [VTQD_RegenTqLimitEn_flg]
  PedalMapWhlTq/4(VTQD_SlideRegenLimTq_Nm) -> [VTQD_SlideRegenLimTq_Nm]
  [BSCPIn_outputs] -> "Rock Mode torque "/1(BSCPIn_outputs)
  [BSignalConvert_outputs] -> "Rock Mode torque "/2(BSignalConvert_outputs)
  [BFunction_outputs] -> "Rock Mode torque "/3(BFunction_outputs)
  "Rock Mode torque "/3(VTQD_RockModePedTq_Nm) -> [VTQD_RockModePedTq_Nm]
  "Rock Mode torque "/4(VTQD_RockModeTqLim_flg) -> [VTQD_RockModeTqLim_flg]
  [BSignalConvert_outputs] -> Low speed control/2(BSignalConvert_outputs)
  [BSCPIn_outputs] -> Low speed control/1(BSCPIn_outputs)
  Low speed control/1(VTQD_LoSpdBrkCtrl_flg) -> [VTQD_LoSpdBrkCtrl_flg]
  [BSignalConvert_outputs] -> Preload system/2(BSignalConvert_outputs)
  [BSCPIn_outputs] -> Preload system/1(BSCPIn_outputs)
  [BFunction_outputs] -> Preload system/3(BFunction_outputs)
  Preload system/1(VTQD_PreLoadHold_flg) -> [VTQD_PreLoadHold_flg]
  Preload system/2(VTQD_PreLoadPreEn_flg) -> [VTQD_PreLoadPreEn_flg]
  [VTQD_CreepEnable_flg] -> Preload system/4(VTQD_CreepEnable_flg)
  Preload system/3(VTQD_PreloadTq_Nm) -> [VTQD_PreloadTq_Nm]
  Preload system/4(VTQD_FrPreloadTq_Nm) -> [VTQD_FrPreloadTq_Nm]
  Preload system/5(VTQD_RrPreloadTq_Nm) -> [VTQD_RrPreloadTq_Nm]
  "Rock Mode torque "/2(VTQD_RockModeTCSReq_flg) -> [VTQD_RockModeTCSReq_flg]
  "Rock Mode torque "/1(VTQD_IVIRockModeEn_flg) -> [VTQD_IVIRockModeEn_flg]
  [VTQD_IVIRockModeEn_flg] -> Driver mode determination/6(VTQD_IVIRockModeEn_flg)
  [BFunction_outputs] -> PedalMapWhlTq/7(BFunction_outputs)
  BMain_outputs/1 -> [BMain_outputs]
  [BMain_outputs] -> PedalMapWhlTq/6(BMain_outputs)
  [VTQD_RollRegenEnable_flg] -> VTQD_RollRegenEnable_flg/1
  [VTQD_BOSEnable_flg] -> VTQD_BOSEnable_flg/1
  [VTQD_BOSTq_Nm] -> VTQD_BOSTq_Nm/1
  [VTQD_IVIRockModeEn_flg] -> VTQD_IVIRockModeEn_flg/1
  [VTQD_LoSpdBrkCtrl_flg] -> VTQD_LoSpdBrkCtrl_flg/1
  [VTQD_RockModeTCSReq_flg] -> VTQD_RockModeTCSReq_flg/1
  [VTQD_RockModePedTq_Nm] -> VTQD_RockModePedTq_Nm/1
  [VTQD_RockModeTqLim_flg] -> VTQD_RockModeTqLim_flg/1
  [VTQD_PreLoadPreEn_flg] -> VTQD_PreLoadPreEn_flg/1
  [VTQD_PreloadTq_Nm] -> VTQD_PreloadTq_Nm/1
  [VTQD_PreLoadHold_flg] -> VTQD_PreLoadHold_flg/1
  [VTQD_CreepWhlTqDem_Nm] -> VTQD_CreepWhlTqDem_Nm/1
  [VTQD_CreepPrLoadEnable_flg] -> VTQD_CreepPrLoadEnable_flg/1
  [VTQD_CreepProtTqEn_flg] -> VTQD_CreepProtTqEn_flg/1
  [VTQD_PedalMapWhlTq_Nm] -> VTQD_PedalMapWhlTq_Nm/1
  [VTQD_EVDriveModeValid_flg] -> VTQD_EVDriveModeValid_flg/1
  [VTQD_RegenTqLimitEn_flg] -> VTQD_RegenTqLimitEn_flg/1
  [VTQD_PedAccTqEn_flg] -> VTQD_PedAccTqEn_flg/1
  [VTQD_SlideRegenLimTq_Nm] -> VTQD_SlideRegenLimTq_Nm/1
  [VTQD_OPDOn2Off_flg] -> VTQD_OPDOn2Off_flg/1
  [VTQD_CreepTCSActive_flg] -> VTQD_CreepTCSActive_flg/1
  [VTQD_RrPreloadTq_Nm] -> VTQD_RrPreloadTq_Nm/1
  [VTQD_FrPreloadTq_Nm] -> VTQD_FrPreloadTq_Nm/1
  [VTQD_CreepEnable_flg] -> VTQD_CreepEnable_flg/1
  [VTQD_CreepBaseTqD_Nm] -> VTQD_CreepBaseTqD_Nm/1
  [VTQD_TqSourceFr_enum] -> RollingRegenJudge/3(VTQD_TqSourceFr_enum)
  [VTQD_TqSourceRr_enum] -> RollingRegenJudge/4(VTQD_TqSourceRr_enum)
  VTQD_TqSourceFr_enum/1 -> [VTQD_TqSourceFr_enum]
  VTQD_TqSourceRr_enum/1 -> [VTQD_TqSourceRr_enum]
  VTQR_FShaftSpdTqLimLow_flg/1 -> [VTQR_FShaftSpdTqLimLow_flg]
  VTQR_FTimerTqLimLow_flg/1 -> [VTQR_FTimerTqLimLow_flg]
  VTQR_RShaftSpdTqLimLow_flg/1 -> [VTQR_RShaftSpdTqLimLow_flg]
  VTQR_RTimerTqLimLow_flg/1 -> [VTQR_RTimerTqLimLow_flg]
  [VTQR_FShaftSpdTqLimLow_flg] -> "Rock Mode torque "/4(VTQR_FShaftSpdTqLimLow_flg)
  [VTQR_FTimerTqLimLow_flg] -> "Rock Mode torque "/5(VTQR_FTimerTqLimLow_flg)
  [VTQR_RShaftSpdTqLimLow_flg] -> "Rock Mode torque "/6(VTQR_RShaftSpdTqLimLow_flg)
  [VTQR_RTimerTqLimLow_flg] -> "Rock Mode torque "/7(VTQR_RTimerTqLimLow_flg)

== system tqdtqr_rebuild_V3/Input_Convert/Main function/Front//Rear EDU Tq Up//Low Limit ==
  note: Rear
  note: Front
  BSCPIn_outputs : Inport
  BSignalConvert_outputs : Inport  Port=2
  BFunction_outputs : Inport  Port=3
  VTQD_WhlTqCapMotFr_Nm : Inport  Port=4
  VTQD_WhlTqCapMotRr_Nm : Inport  Port=5
  VTQD_WhlTqCapGenFr_Nm : Inport  Port=6
  VTQD_WhlTqCapGenRr_Nm : Inport  Port=7
  AND{,1..2,4,18..21} (8 alike) : Logic  AllPortsSameDT=off  OutDataTypeStr=boolean
  Bus Selector : BusSelector  OutputSignals=VTQD_RDCActive_enum,VINP_FrntAxlTrqReqDrv_Nm,VINP_FrPTCSActive_flg,VINP_RearAxlTrqReqDrv_Nm,VINP_RrPTCSActive_flg
  Bus Selector1 : BusSelector  OutputSignals=VTQR_RampTqCMDGain_c
  Bus Selector2 : BusSelector  OutputSignals=VTQD_GearActualPosn_enum
  Constant{6,11,18,28} (4 alike) : Constant  Value=ENUM_CANRDCACTSTA_EXITIMMEDIATELY
  Constant{16,20,24,26} (4 alike) : Constant  Value=KTQR_NewRampArchSW_flg
  Constant{17,21,25,27} (4 alike) : Constant  Value=ENUM_GEARACTUALPOSN_R
  Constant{7..8,19,29} (4 alike) : Constant  Value=ZERO_FLOAT
  Constant{42..44,46} (4 alike) : Constant  Value=ENUM_GEARACTUALPOSN_D
  Constant45 : Constant  Value=KTQR_FinalFEDUTrqLowLim_Nm
  Constant47 : Constant  Value=KTQR_FinalFEDUTrqUpLim_Nm
  Equal{,1..7} (8 alike) : RelationalOperator  Operator===  OutDataTypeStr=boolean  RndMeth=Simplest
  Equal{10..13} (4 alike) : RelationalOperator  Operator=~=  OutDataTypeStr=boolean  RndMeth=Simplest
  Min : MinMax  Inputs=2
  Min1 : MinMax  Function=max  Inputs=2
  Min2 : MinMax  Inputs=2
  Min3 : MinMax  Function=max  Inputs=2
  Product{3..4,6..7} (4 alike) : Product
  RegenLV_inc1 : Constant  Value=KTQR_FinalFEDUTrqLowLim_Nm  OutDataTypeStr=single
  RegenLV_inc{9..12} (4 alike) : Constant  Value=KTQR_TCSActTQRLimSW_flg  OutDataTypeStr=single
  RegenLV_inc13 : Constant  Value=KTQR_FinalREDUTrqUpLim_Nm  OutDataTypeStr=single
  RegenLV_inc14 : Constant  Value=KTQR_FinalREDUTrqLowLim_Nm  OutDataTypeStr=single
  RegenLV_inc2 : Constant  Value=KTQR_FinalFEDUTrqUpLim_Nm  OutDataTypeStr=single
  RegenLV_inc3 : Constant  Value=KTQR_FinalREDUTrqLowLim_Nm  OutDataTypeStr=single
  RegenLV_inc4 : Constant  Value=KTQR_FinalREDUTrqUpLim_Nm  OutDataTypeStr=single
  RegenLV_inc5 : Constant  Value=KTQR_FinalFEDUTrqUpLim_Nm  OutDataTypeStr=single
  RegenLV_inc6 : Constant  Value=KTQR_FinalFEDUTrqLowLim_Nm  OutDataTypeStr=single
  RegenLV_inc7 : Constant  Value=KTQR_FinalREDUTrqUpLim_Nm  OutDataTypeStr=single
  RegenLV_inc8 : Constant  Value=KTQR_FinalREDUTrqLowLim_Nm  OutDataTypeStr=single
  Switch{6..9,13..16,18..21,28..31} (16 alike) : Switch  Criteria=u2 ~= 0
      settings: AttributesFormatString=%<Criteria>
  VTQR_ActFEDUTqLowLimit_Nm : Outport
  VTQR_ActFEDUTqUpLimit_Nm : Outport  Port=2
  VTQR_ActREDUTqUpLimit_Nm : Outport  Port=3
  VTQR_ActREDUTqLowLimit_Nm : Outport  Port=4
  wires:
  [VTQD_GearActualPosn_enum] -> Equal3/1
  Switch8/1 -> Switch16/3
  Constant20/1 -> AND1/2
  Constant19/1 -> Switch15/1
  AND1/1 -> Switch16/2
  Product4/1 -> Switch16/1
  [VTQD_RDCActive_enum] -> Equal2/1
  [VINP_FrntAxlTrqReqDrv_Nm] -> Switch8/1
  Min/1 -> [VTQR_ActFEDUTqUpLimit_Nm]  "VTQR_ActFEDUTqUpLimit_Nm"
  [VTQD_GearActualPosn_enum] -> Equal13/1
  RegenLV_inc2/1 -> Switch8/3
  Constant18/1 -> Equal2/2
  Equal2/1 -> Switch15/2
  Switch15/1 -> Product4/2
  Constant46/1 -> Equal13/2
  RegenLV_inc6/1 -> Switch15/3
  Constant21/1 -> Equal3/2
  RegenLV_inc9/1 -> AND18/2
  AND18/1 -> Switch8/2
  [VTQR_RampTqCMDGain_c] -> Product4/1
  Switch16/1 -> Min/1
  [VINP_FrPTCSActive_flg] -> AND18/1
  Switch31/1 -> Min/2
  [VTQD_WhlTqCapMotFr_Nm] -> Switch31/3
  Constant47/1 -> Switch31/1
  Equal3/1 -> AND1/1
  Equal13/1 -> Switch31/2
  RegenLV_inc1/1 -> Switch6/3
  [VTQR_RampTqCMDGain_c] -> Product3/1
  Switch14/1 -> Product3/2
  [VTQD_GearActualPosn_enum] -> Equal1/1
  [VINP_FrntAxlTrqReqDrv_Nm] -> Switch14/1
  Switch6/1 -> Switch13/3
  RegenLV_inc5/1 -> Switch14/3
  Switch30/1 -> Min1/2
  [VINP_FrPTCSActive_flg] -> AND19/1
  [VTQD_WhlTqCapGenFr_Nm] -> Switch30/3
  Constant44/1 -> Equal12/2
  Product3/1 -> Switch13/1
  Equal12/1 -> Switch30/2
  Constant45/1 -> Switch30/1
  [VTQD_GearActualPosn_enum] -> Equal12/1
  AND/1 -> Switch13/2
  Equal1/1 -> AND/1
  Switch13/1 -> Min1/1
  RegenLV_inc10/1 -> AND19/2
  Constant6/1 -> Equal/2
  Constant7/1 -> Switch6/1
  AND19/1 -> Switch14/2
  Equal/1 -> Switch6/2
  Constant17/1 -> Equal1/2
  [VTQD_RDCActive_enum] -> Equal/1
  Min1/1 -> [VTQR_ActFEDUTqLowLimit_Nm]  "VTQR_ActFEDUTqLowLimit_Nm"
  Constant16/1 -> AND/2
  RegenLV_inc4/1 -> Switch9/3
  RegenLV_inc13/1 -> Switch28/1
  Constant42/1 -> Equal10/2
  AND21/1 -> Switch9/2
  Equal10/1 -> Switch28/2
  [VTQD_WhlTqCapMotRr_Nm] -> Switch28/3
  Switch28/1 -> Min2/2
  Constant26/1 -> AND4/2
  [VINP_RrPTCSActive_flg] -> AND21/1
  Equal6/1 -> AND4/1
  [VTQR_RampTqCMDGain_c] -> Product7/1
  Constant27/1 -> Equal6/2
  Equal7/1 -> Switch21/2
  [VTQD_RDCActive_enum] -> Equal7/1
  RegenLV_inc8/1 -> Switch21/3
  AND4/1 -> Switch20/2
  Switch21/1 -> Product7/2
  Switch9/1 -> Switch20/3
  Constant28/1 -> Equal7/2
  Min2/1 -> [VTQR_ActREDUTqUpLimit_Nm]  "VTQR_ActREDUTqUpLimit_Nm"
  Product7/1 -> Switch20/1
  Constant29/1 -> Switch21/1
  Switch20/1 -> Min2/1
  [VTQD_GearActualPosn_enum] -> Equal10/1
  [VTQD_GearActualPosn_enum] -> Equal6/1
  [VINP_RearAxlTrqReqDrv_Nm] -> Switch9/1
  RegenLV_inc12/1 -> AND21/2
  RegenLV_inc7/1 -> Switch19/3
  Switch7/1 -> Switch18/3
  Switch19/1 -> Product6/2
  [VTQD_GearActualPosn_enum] -> Equal5/1
  Product6/1 -> Switch18/1
  Constant8/1 -> Switch7/1
  [VTQD_RDCActive_enum] -> Equal4/1
  Equal4/1 -> Switch7/2
  Constant11/1 -> Equal4/2
  [VINP_RrPTCSActive_flg] -> AND20/1
  Equal5/1 -> AND2/1
  RegenLV_inc3/1 -> Switch7/3
  AND20/1 -> Switch19/2
  Constant43/1 -> Equal11/2
  [VTQD_WhlTqCapGenRr_Nm] -> Switch29/3
  Min3/1 -> [VTQR_ActREDUTqLowLimit_Nm]  "VTQR_ActREDUTqLowLimit_Nm"
  Switch29/1 -> Min3/2
  Equal11/1 -> Switch29/2
  RegenLV_inc14/1 -> Switch29/1
  Constant25/1 -> Equal5/2
  AND2/1 -> Switch18/2
  Constant24/1 -> AND2/2
  RegenLV_inc11/1 -> AND20/2
  [VTQR_RampTqCMDGain_c] -> Product6/1
  Switch18/1 -> Min3/1
  [VTQD_GearActualPosn_enum] -> Equal11/1
  [VINP_RearAxlTrqReqDrv_Nm] -> Switch19/1
  BSCPIn_outputs/1 -> Bus Selector/1
  BSignalConvert_outputs/1 -> Bus Selector1/1
  BFunction_outputs/1 -> Bus Selector2/1
  Bus Selector/1 -> [VTQD_RDCActive_enum]  "<VTQD_RDCActive_enum>"
  Bus Selector/2 -> [VINP_FrntAxlTrqReqDrv_Nm]  "<VINP_FrntAxlTrqReqDrv_Nm>"
  Bus Selector/3 -> [VINP_FrPTCSActive_flg]  "<VINP_FrPTCSActive_flg>"
  Bus Selector1/1 -> [VTQR_RampTqCMDGain_c]  "<VTQR_RampTqCMDGain_c>"
  Bus Selector2/1 -> [VTQD_GearActualPosn_enum]  "<VTQD_GearActualPosn_enum>"
  VTQD_WhlTqCapMotFr_Nm/1 -> [VTQD_WhlTqCapMotFr_Nm]
  VTQD_WhlTqCapGenFr_Nm/1 -> [VTQD_WhlTqCapGenFr_Nm]
  Bus Selector/4 -> [VINP_RearAxlTrqReqDrv_Nm]  "<VINP_RearAxlTrqReqDrv_Nm>"
  Bus Selector/5 -> [VINP_RrPTCSActive_flg]  "<VINP_RrPTCSActive_flg>"
  VTQD_WhlTqCapMotRr_Nm/1 -> [VTQD_WhlTqCapMotRr_Nm]
  VTQD_WhlTqCapGenRr_Nm/1 -> [VTQD_WhlTqCapGenRr_Nm]
  [VTQR_ActFEDUTqLowLimit_Nm] -> VTQR_ActFEDUTqLowLimit_Nm/1
  [VTQR_ActFEDUTqUpLimit_Nm] -> VTQR_ActFEDUTqUpLimit_Nm/1
  [VTQR_ActREDUTqUpLimit_Nm] -> VTQR_ActREDUTqUpLimit_Nm/1
  [VTQR_ActREDUTqLowLimit_Nm] -> VTQR_ActREDUTqLowLimit_Nm/1
